simulink model "Copy_of_VTOLTiltrotor"  (R2024a)
settings: configuration reference "VTOLConfiguration" (kept outside this file)
undefined symbols (not defined in the file): airspeed, Battery, BCE12, BCE_Set_init, BMS_Controller_State, C, Cell10_P, Cell11_P, Cell12_P, Cell1_N, Cell1_P, Cell2_P, Cell3_P, Cell4_P, Cell5_P, Cell6_P, Cell7_P, Cell8_P, Cell9_P, Cell_Temperatures, Cell_Voltages, Charging_State, CityMission, control, controlParams, ControlSampleTime, CriticalTiltAngle, currentFactor, CV_Gain, ddx, ddy, ddz, Device_01, DiscIntNeverNeededParam, dx, dy, dz, Earth, env, F, F28379D_ADC_MaxCount, F28379D_ADC_Vmax, FixedWingMission, flightState, Foc_Ki_IxTcpu, Foc_Ki_S, Foc_Kp_I, Foc_Kp_S, fractalcoef, FSState, FWControlParams, HoverMission, I_cc, Ia_offset, Ib_offset, iniRoll, initPitch, iniYaw, IO334, IO334_DAC_Vmax ... (+55)
libraries: slrealtimeethercatlib x109, simulink x81, fl_lib x65, slpidlib x49, mcbcontrolslib x48, nesl_utility x43, speedgoatlib_hdlCoder_IO3xx x31, canmsglib x17, slrealtimeutilitieslib x13, mcbhdlplantlib x13, speedgoatlib_IO611 x12, dspstat3 x12
(part 1 of 20)
settings Model: DataDictionary=VTOLDynamicsData.sldd  Creator=The MathWorks, Inc.  LastModifiedBy=jatin.anand
settings ConfigSetRef: SourceName=VTOLConfiguration

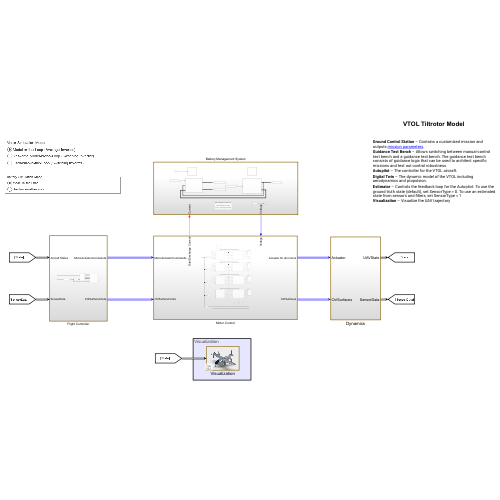
[thumbnail: Simulink's stored preview of the top-level diagram]
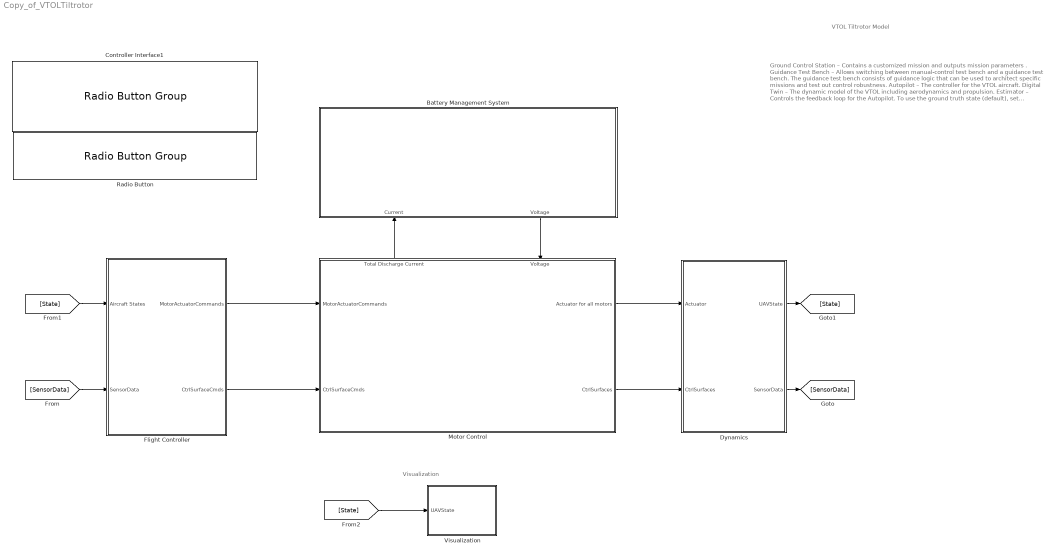
== system Copy_of_VTOLTiltrotor ==
  note: Ground Control Station – Contains a customized mission and outputs mission parameters .
      | Guidance Test Bench – Allows switching between manual-control test bench and a guidance test bench. The guidance test bench consists of guidance logic that can be used to architect specific missions and test out control robustness.
      | Autopilot – The controller for the VTOL aircraft.
      | Digital Twin – The dynamic model of the VTOL including aerodynamics and propulsion.
      | Estimator – Controls the feedback loop for the Autopilot. To use the ground truth state (default), set SensorType = 0. To use an estimated state from sensors and filters, set SensorType = 1
      | Visualization – Visualize the UAV trajectory
  note: VTOL Tiltrotor Model
  note: Visualization
  Battery Management System : Subsystem
      settings: PortSchema="{\"entries\":[{\"content\":{\"sides\":[{\"content\":{},\"type\":\"ConnectorPlacement.EquallySpacedRectSide\",\"uuid\":\"ad4822d7-5628-4510-88b7-b705ff74b914\"},{\"content\":{\"side\":\"RIGHT\"},\"type\":\"ConnectorPlacement.EquallySpacedRectSide\",\"uuid\":\"08045353-b32a-4841-afa7-c31ec693f3bd\"},{\"content\":{\"side\":\"TOP\"},\"type\":\"ConnectorPlacement.EquallySpacedRectSide\",\"uuid\":\"6a6533a3-371c-43cc-ab21-2cdd93971ace\"},{\"content\":{\"connectorIds\":[\"In1\",\"Out1\"],\"side\":\"BOTTOM\"},\"type\":\"ConnectorPlacement.EquallySpacedRectSide\",\"uuid\":\"23933915-aea2-4276-b64d-d3fc5163d9da\"}]},\"type\":\"ConnectorPlacement.EquallySpacedConnector\",\"uuid\":\"ad7e7a57-8abd-4902-b93b-ccdedcf72dce\"}],\"packageUris\":[\"http://schema.mathworks.com/mf0/Connector/R2020b\"],\"version\":\"1.0\"}"
  Controller Interface1 : RadioButtonGroup  LabelPosition=Hide  SelectedLabel=Model-in-the-Loop (Average Inverter)  ButtonGroupName=Motor Simulation Mode
      settings: Values={{'Model-in-the-Loop (Average Inverter)', 'Real-time Model-in-the-Loop (Switching Inverter)', 'Hardware-in-the-Loop (Switching Inverter)'}, [1 2 3]}
  Dynamics : Subsystem
  Flight Controller : Subsystem
  Motor Control : Subsystem
      settings: PortSchema="{\"entries\":[{\"content\":{\"sides\":[{\"content\":{\"connectorIds\":[\"In1\",\"In2\"]},\"type\":\"ConnectorPlacement.EquallySpacedRectSide\",\"uuid\":\"94b5e33d-15f7-4229-89dd-c5549510cb9d\"},{\"content\":{\"connectorIds\":[\"Out1\",\"Out2\"],\"side\":\"RIGHT\"},\"type\":\"ConnectorPlacement.EquallySpacedRectSide\",\"uuid\":\"879591cf-6d91-4a7e-b358-28ad8026a1fe\"},{\"content\":{\"connectorIds\":[\"Out3\",\"In3\"],\"side\":\"TOP\"},\"type\":\"ConnectorPlacement.EquallySpacedRectSide\",\"uuid\":\"fed77af4-f074-449a-8fce-c96eeb48edb7\"}]},\"type\":\"ConnectorPlacement.EquallySpacedConnector\",\"uuid\":\"f2702da8-edb1-45fe-ba32-a4867476937a\"}],\"packageUris\":[\"http://schema.mathworks.com/mf0/Connector/R2020b\"],\"version\":\"1.0\"}"
  Radio Button : RadioButtonGroup  LabelPosition=Hide  SelectedLabel=Model-in-the-Loop  ButtonGroupName=Battery Simulation Mode
      settings: Values={{'Model-in-the-Loop', 'Hardware-in-the-Loop'}, [0 1]}
  Visualization : Subsystem  Variant=on  VariantControl=Visualization
      mask Display: image('TiltrotorVisualization.PNG'); % Use "Edit Image" on toolstrip to change.
  wires:
  Dynamics/2(SensorData) -> [SensorData]
  Dynamics/1(UAVState) -> [State]
  [SensorData] -> Flight Controller/2(SensorData)
  [State] -> Flight Controller/1(Aircraft States)
  [State] -> Visualization/1(UAVState)
  Flight Controller/1(MotorActuatorCommands) -> Motor Control/1(MotorActuatorCommands)
  Flight Controller/2(CtrlSurfaceCmds) -> Motor Control/2(CtrlSurfaceCmds)
  Motor Control/1(Actuator for all motors) -> Dynamics/1(Actuator)
  Motor Control/2(CtrlSurfaces) -> Dynamics/2(CtrlSurfaces)
  Motor Control/3(Total Discharge Current) -> Battery Management System/1(Current)
  Battery Management System/1(Voltage) -> Motor Control/3(Voltage)

== system Copy_of_VTOLTiltrotor/Battery Management System ==
  note: Battery Management System HIL
      |
      | Reference application model
      | © 2007 - 2024 Speedgoat GmbH
  Current : Inport
  BMS : Subsystem  Variant=on  VariantControl=Choice
      mask Display: image('BMS.png'); % Use "Edit Image" on toolstrip to change.
  Battery : Subsystem
      mask Display: image('battery.png'); % Use "Edit Image" on toolstrip to change.
  Instrumentation : Subsystem
      mask Display: image('tunable.png'); % Use "Edit Image" on toolstrip to change.
  User Interface : Subsystem
      mask Display: image('UI.png'); % Use "Edit Image" on toolstrip to change.
  Voltage : Outport
  tag scope: Controller_Info=global, Controller_Output=global, Sensor_Values=global
  wires:
  [Current_Request] -> Battery/1(Current_Request)
  BMS/1(Controller_Info) -> [Controller_Info]  "Controller_Info"
  Battery/1(Sensor_Values) -> [Sensor_Values], BMS/2(Sensor_Values)
  [State_Request] -> BMS/1(State_Request)
  BMS/2(Controller_Output) -> [Controller_Output]  "Controller_Output"
  Current/1 -> Instrumentation/1(Current)
  [Voltage] -> Voltage/1
  connections:
  Battery/RConn1 -- BMS/LConn1

== system Copy_of_VTOLTiltrotor/Dynamics ==
  note: Forces and Moments - VTOL UAV plant model and weather model
      | 6DOF (Euler Angles Conversion) - Converts forces and moments from body to inertial frame
      | Ground Truth Bus - converts UAV States into bus
  Actuator : Inport
  CtrlSurfaces : Inport  Port=2
  6DOF (Euler Angles)1 : shared6dof/6DOF (Euler Angles)  units=Metric (MKS)  mtype=Fixed  rep=Euler Angles  xme_0=[xGround, yGround, zGround]  Vm_0=[vIni 0 0]  eul_0=[iniRoll initPitch iniYaw]  pm_0=[0 0 0]  mass_0=6.031  mass_e=0.5  mass_f=2.0  inertia=[uavParam.geom.Ixx 0 0; 0 uavParam.geom.Iyy 0; 0 0 uavParam.geom.Izz]  inertia_e=eye(3)  inertia_f=2*eye(3)  k_quat=1.0  vre_flag=on  abi_flag=on  aMode=0  xme_statename=''  Vm_statename=''  eul_statename=''  quat_statename=''  pm_statename=''  mass_statename=''
  Bus Selector : BusSelector  OutputSignals=RotorParameters.w1,RotorParameters.w2,RotorParameters.w3,RotorParameters.w4
  Force and Moments : Subsystem
  Ground Truth Bus : Subsystem
  Scope : Scope  NumInputPorts=4
  Terminator : Terminator
  Variant Subsystem : Subsystem  Variant=on  VariantControl=Choice
  UAVState : Outport
  SensorData : Outport  Port=2
  wires:
  Force and Moments/1(F) -> 6DOF (Euler Angles)1/1
  Force and Moments/2(M) -> 6DOF (Euler Angles)1/2
  Actuator/1 -> Force and Moments/1(Actuator)
  CtrlSurfaces/1 -> Force and Moments/2(CtrlSurfaces)
  6DOF (Euler Angles)1/1 -> Ground Truth Bus/1(Ve)  "Ve"
  6DOF (Euler Angles)1/2 -> Ground Truth Bus/2(Xe)  "Xe"
  6DOF (Euler Angles)1/3 -> Ground Truth Bus/3(Euler)  "Euler"
  6DOF (Euler Angles)1/4 -> Ground Truth Bus/4(DCMbe)  "DCMbe"
  6DOF (Euler Angles)1/5 -> Ground Truth Bus/5(Vb)  "Vb"
  6DOF (Euler Angles)1/6 -> Ground Truth Bus/6(pqr)  "pqr"
  6DOF (Euler Angles)1/7 -> Terminator/1
  6DOF (Euler Angles)1/8 -> Ground Truth Bus/7(Abb)  "Abb"
  Force and Moments/3(RotorParams) -> Ground Truth Bus/9(RotorParams)  "RotorParams"
  Force and Moments/4(AirData) -> Ground Truth Bus/10(AirData)
  Variant Subsystem/1(SensorData) -> SensorData/1
  6DOF (Euler Angles)1/9 -> Ground Truth Bus/8(Abe)
  Ground Truth Bus/1(Ground Truth) -> Bus Selector/1, UAVState/1, Force and Moments/3(States), Variant Subsystem/1(UAVStates)  "Ground Truth"
  Bus Selector/1 -> Scope/1  "<w1>"
  Bus Selector/2 -> Scope/2  "<w2>"
  Bus Selector/3 -> Scope/3  "<w3>"
  Bus Selector/4 -> Scope/4  "<w4>"

== system Copy_of_VTOLTiltrotor/Flight Controller ==
  Aircraft States : Inport
  SensorData : Inport  Port=2
  Autopilot : Subsystem
  Estimator : Subsystem  Variant=on
  Ground Control Station : Subsystem
  Guidance Test Bench : Subsystem
  MotorActuatorCommands : Outport
  CtrlSurfaceCmds : Outport  Port=2
  wires:
  Guidance Test Bench/3(AACSP) -> Autopilot/3(AAC)
  Estimator/1(EstimatedStates) -> Autopilot/6(EstimatedStates), Ground Control Station/1(UAVState)
  Ground Control Station/1(Global Mission) -> Guidance Test Bench/2(Global Mission)
  Guidance Test Bench/5(FlightMode) -> Autopilot/5(FlightMode)
  Guidance Test Bench/1(HoverSP) -> Autopilot/1(HoverCommands)
  Guidance Test Bench/2(FixedWingSP) -> Autopilot/2(FixedWingSP)
  SensorData/1 -> Estimator/1(SensorData)
  Guidance Test Bench/4(ctrlMode) -> Autopilot/4(CtrlMode)
  Autopilot/1(MotorActuatorCommands) -> MotorActuatorCommands/1
  Autopilot/2(CtrlSurfaceCmds) -> CtrlSurfaceCmds/1
  Aircraft States/1 -> Guidance Test Bench/1(Aircraft States)

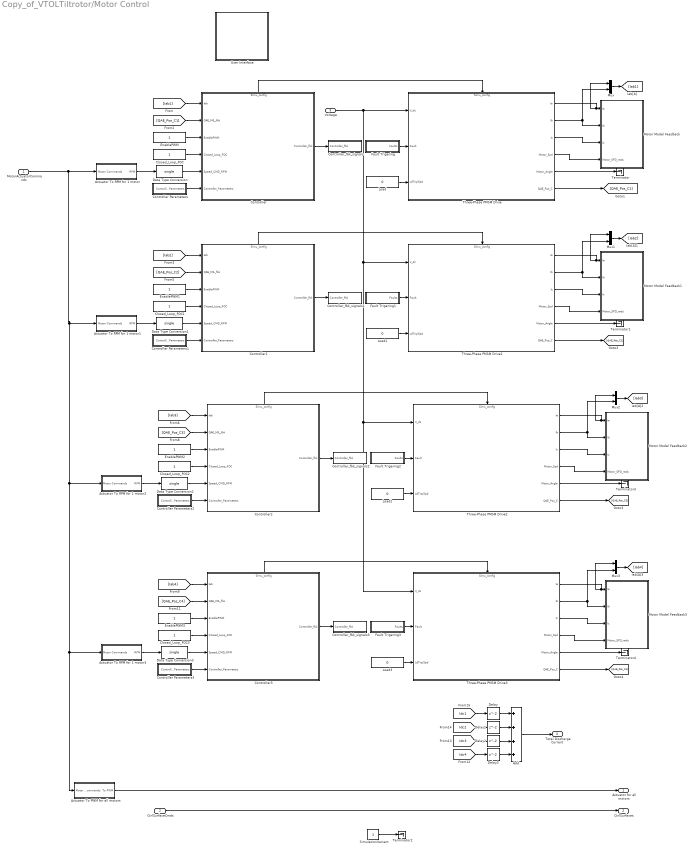
== system Copy_of_VTOLTiltrotor/Motor Control ==
  MotorActuatorCommands : Inport
  CtrlSurfaceCmds : Inport  Port=2
  Voltage : Inport  Port=3
  Actuator To PWM for all motors : Subsystem
  Actuator To RPM for 1 motor : Subsystem
  Actuator To RPM for 1 motor1 : Subsystem
  Actuator To RPM for 1 motor2 : Subsystem
  Actuator To RPM for 1 motor3 : Subsystem
  Add : Sum  Inputs=++++
  Closed_Loop_FOC{,1..3} (4 alike) : Constant  OutDataTypeStr=boolean  SampleTime=Ts_UI
  Controller : Subsystem  Variant=on  VariantControl=Choice
      settings: PortSchema="{\"entries\":[{\"content\":{\"sides\":[{\"content\":{\"connectorIds\":[\"In1\",\"In2\",\"In3\",\"In4\",\"In5\",\"In6\"]},\"type\":\"ConnectorPlacement.EquallySpacedRectSide\",\"uuid\":\"39f08c92-b87f-4f95-877f-fef0e466fbdb\"},{\"content\":{\"connectorIds\":[\"Out1\"],\"side\":\"RIGHT\"},\"type\":\"ConnectorPlacement.EquallySpacedRectSide\",\"uuid\":\"6fadd6f2-7db3-41c1-89a7-be1692c18c49\"},{\"content\":{\"connectorIds\":[\"Out2\"],\"side\":\"TOP\"},\"type\":\"ConnectorPlacement.EquallySpacedRectSide\",\"uuid\":\"aea4ee68-7094-4bdc-b416-2d8969306971\"}]},\"type\":\"ConnectorPlacement.EquallySpacedConnector\",\"uuid\":\"e129f01f-1291-4735-8ea4-164650c1b4f8\"}],\"packageUris\":[\"http://schema.mathworks.com/mf0/Connector/R2020b\"],\"version\":\"1.0\"}"
      mask Display: image('MCUMask.png');
  Controller Parameters : Subsystem
  Controller Parameters1 : Subsystem
  Controller Parameters2 : Subsystem
  Controller Parameters3 : Subsystem
  Controller1 : Subsystem  Variant=on  VariantControl=Choice
      settings: PortSchema="{\"entries\":[{\"content\":{\"sides\":[{\"content\":{\"connectorIds\":[\"In1\",\"In2\",\"In3\",\"In4\",\"In5\",\"In6\"]},\"type\":\"ConnectorPlacement.EquallySpacedRectSide\",\"uuid\":\"39f08c92-b87f-4f95-877f-fef0e466fbdb\"},{\"content\":{\"connectorIds\":[\"Out1\"],\"side\":\"RIGHT\"},\"type\":\"ConnectorPlacement.EquallySpacedRectSide\",\"uuid\":\"6fadd6f2-7db3-41c1-89a7-be1692c18c49\"},{\"content\":{\"connectorIds\":[\"Out2\"],\"side\":\"TOP\"},\"type\":\"ConnectorPlacement.EquallySpacedRectSide\",\"uuid\":\"aea4ee68-7094-4bdc-b416-2d8969306971\"}]},\"type\":\"ConnectorPlacement.EquallySpacedConnector\",\"uuid\":\"e129f01f-1291-4735-8ea4-164650c1b4f8\"}],\"packageUris\":[\"http://schema.mathworks.com/mf0/Connector/R2020b\"],\"version\":\"1.0\"}"
      mask Display: image('MCUMask.png');
  Controller2 : Subsystem  Variant=on  VariantControl=Choice
      settings: PortSchema="{\"entries\":[{\"content\":{\"sides\":[{\"content\":{\"connectorIds\":[\"In1\",\"In2\",\"In3\",\"In4\",\"In5\",\"In6\"]},\"type\":\"ConnectorPlacement.EquallySpacedRectSide\",\"uuid\":\"39f08c92-b87f-4f95-877f-fef0e466fbdb\"},{\"content\":{\"connectorIds\":[\"Out1\"],\"side\":\"RIGHT\"},\"type\":\"ConnectorPlacement.EquallySpacedRectSide\",\"uuid\":\"6fadd6f2-7db3-41c1-89a7-be1692c18c49\"},{\"content\":{\"connectorIds\":[\"Out2\"],\"side\":\"TOP\"},\"type\":\"ConnectorPlacement.EquallySpacedRectSide\",\"uuid\":\"aea4ee68-7094-4bdc-b416-2d8969306971\"}]},\"type\":\"ConnectorPlacement.EquallySpacedConnector\",\"uuid\":\"e129f01f-1291-4735-8ea4-164650c1b4f8\"}],\"packageUris\":[\"http://schema.mathworks.com/mf0/Connector/R2020b\"],\"version\":\"1.0\"}"
      mask Display: image('MCUMask.png');
  Controller3 : Subsystem  Variant=on  VariantControl=Choice
      settings: PortSchema="{\"entries\":[{\"content\":{\"sides\":[{\"content\":{\"connectorIds\":[\"In1\",\"In2\",\"In3\",\"In4\",\"In5\",\"In6\"]},\"type\":\"ConnectorPlacement.EquallySpacedRectSide\",\"uuid\":\"39f08c92-b87f-4f95-877f-fef0e466fbdb\"},{\"content\":{\"connectorIds\":[\"Out1\"],\"side\":\"RIGHT\"},\"type\":\"ConnectorPlacement.EquallySpacedRectSide\",\"uuid\":\"6fadd6f2-7db3-41c1-89a7-be1692c18c49\"},{\"content\":{\"connectorIds\":[\"Out2\"],\"side\":\"TOP\"},\"type\":\"ConnectorPlacement.EquallySpacedRectSide\",\"uuid\":\"aea4ee68-7094-4bdc-b416-2d8969306971\"}]},\"type\":\"ConnectorPlacement.EquallySpacedConnector\",\"uuid\":\"e129f01f-1291-4735-8ea4-164650c1b4f8\"}],\"packageUris\":[\"http://schema.mathworks.com/mf0/Connector/R2020b\"],\"version\":\"1.0\"}"
      mask Display: image('MCUMask.png');
  Controller_fbk_signals : Subsystem
  Controller_fbk_signals1 : Subsystem
  Controller_fbk_signals2 : Subsystem
  Controller_fbk_signals3 : Subsystem
  Data Type Conversion{,1..3} (4 alike) : DataTypeConversion  OutDataTypeStr=single  SaturateOnIntegerOverflow=off  RndMeth=Floor
  Delay{,1..3} (4 alike) : Delay
  EnablePWM{,1..3} (4 alike) : Constant  OutDataTypeStr=boolean  SampleTime=Ts_UI
  Fault Trigering : Subsystem
  Fault Trigering1 : Subsystem
  Fault Trigering2 : Subsystem
  Fault Trigering3 : Subsystem
  Load{,1..3} (4 alike) : Constant  Value=0  OutDataTypeStr=single
  Motor Model Feedback : Subsystem
  Motor Model Feedback1 : Subsystem
  Motor Model Feedback2 : Subsystem
  Motor Model Feedback3 : Subsystem
  Mux{,1..3} (4 alike) : Mux  Inputs=2
  SimulationVariant : Constant
  Terminator{,1..4} (5 alike) : Terminator
  Three-Phase PMSM Drive : Subsystem  Variant=on  VariantControl=Choice
      settings: PortSchema="{\"entries\":[{\"content\":{\"sides\":[{\"content\":{\"connectorIds\":[\"In1\",\"In2\",\"In3\"]},\"type\":\"ConnectorPlacement.EquallySpacedRectSide\",\"uuid\":\"be3bef0c-fa0d-49a9-8d81-4a9438f9f09e\"},{\"content\":{\"connectorIds\":[\"Out1\",\"Out2\",\"Out3\",\"Out4\",\"Out5\",\"Out6\"],\"side\":\"RIGHT\"},\"type\":\"ConnectorPlacement.EquallySpacedRectSide\",\"uuid\":\"a97c4291-bd47-47ae-a87a-e148291abc4a\"},{\"content\":{\"connectorIds\":[\"In4\"],\"side\":\"TOP\"},\"type\":\"ConnectorPlacement.EquallySpacedRectSide\",\"uuid\":\"93bcf0c4-5b44-4ac3-b6c3-6b4577237bd1\"}]},\"type\":\"ConnectorPlacement.EquallySpacedConnector\",\"uuid\":\"9c4ab161-5f4a-4191-8213-47b9045836c1\"}],\"packageUris\":[\"http://schema.mathworks.com/mf0/Connector/R2020b\"],\"version\":\"1.0\"}"
      mask Display: image('pmsmMask.png'); % Use "Edit Image" on toolstrip to change.
  Three-Phase PMSM Drive1 : Subsystem  Variant=on  VariantControl=Choice
      settings: PortSchema="{\"entries\":[{\"content\":{\"sides\":[{\"content\":{\"connectorIds\":[\"In1\",\"In2\",\"In3\"]},\"type\":\"ConnectorPlacement.EquallySpacedRectSide\",\"uuid\":\"be3bef0c-fa0d-49a9-8d81-4a9438f9f09e\"},{\"content\":{\"connectorIds\":[\"Out1\",\"Out2\",\"Out3\",\"Out4\",\"Out5\",\"Out6\"],\"side\":\"RIGHT\"},\"type\":\"ConnectorPlacement.EquallySpacedRectSide\",\"uuid\":\"a97c4291-bd47-47ae-a87a-e148291abc4a\"},{\"content\":{\"connectorIds\":[\"In4\"],\"side\":\"TOP\"},\"type\":\"ConnectorPlacement.EquallySpacedRectSide\",\"uuid\":\"93bcf0c4-5b44-4ac3-b6c3-6b4577237bd1\"}]},\"type\":\"ConnectorPlacement.EquallySpacedConnector\",\"uuid\":\"9c4ab161-5f4a-4191-8213-47b9045836c1\"}],\"packageUris\":[\"http://schema.mathworks.com/mf0/Connector/R2020b\"],\"version\":\"1.0\"}"
      mask Display: image('pmsmMask.png'); % Use "Edit Image" on toolstrip to change.
  Three-Phase PMSM Drive2 : Subsystem  Variant=on  VariantControl=Choice
      settings: PortSchema="{\"entries\":[{\"content\":{\"sides\":[{\"content\":{\"connectorIds\":[\"In1\",\"In2\",\"In3\"]},\"type\":\"ConnectorPlacement.EquallySpacedRectSide\",\"uuid\":\"be3bef0c-fa0d-49a9-8d81-4a9438f9f09e\"},{\"content\":{\"connectorIds\":[\"Out1\",\"Out2\",\"Out3\",\"Out4\",\"Out5\",\"Out6\"],\"side\":\"RIGHT\"},\"type\":\"ConnectorPlacement.EquallySpacedRectSide\",\"uuid\":\"a97c4291-bd47-47ae-a87a-e148291abc4a\"},{\"content\":{\"connectorIds\":[\"In4\"],\"side\":\"TOP\"},\"type\":\"ConnectorPlacement.EquallySpacedRectSide\",\"uuid\":\"93bcf0c4-5b44-4ac3-b6c3-6b4577237bd1\"}]},\"type\":\"ConnectorPlacement.EquallySpacedConnector\",\"uuid\":\"9c4ab161-5f4a-4191-8213-47b9045836c1\"}],\"packageUris\":[\"http://schema.mathworks.com/mf0/Connector/R2020b\"],\"version\":\"1.0\"}"
      mask Display: image('pmsmMask.png'); % Use "Edit Image" on toolstrip to change.
  Three-Phase PMSM Drive3 : Subsystem  Variant=on  VariantControl=Choice
      settings: PortSchema="{\"entries\":[{\"content\":{\"sides\":[{\"content\":{\"connectorIds\":[\"In1\",\"In2\",\"In3\"]},\"type\":\"ConnectorPlacement.EquallySpacedRectSide\",\"uuid\":\"be3bef0c-fa0d-49a9-8d81-4a9438f9f09e\"},{\"content\":{\"connectorIds\":[\"Out1\",\"Out2\",\"Out3\",\"Out4\",\"Out5\",\"Out6\"],\"side\":\"RIGHT\"},\"type\":\"ConnectorPlacement.EquallySpacedRectSide\",\"uuid\":\"a97c4291-bd47-47ae-a87a-e148291abc4a\"},{\"content\":{\"connectorIds\":[\"In4\"],\"side\":\"TOP\"},\"type\":\"ConnectorPlacement.EquallySpacedRectSide\",\"uuid\":\"93bcf0c4-5b44-4ac3-b6c3-6b4577237bd1\"}]},\"type\":\"ConnectorPlacement.EquallySpacedConnector\",\"uuid\":\"9c4ab161-5f4a-4191-8213-47b9045836c1\"}],\"packageUris\":[\"http://schema.mathworks.com/mf0/Connector/R2020b\"],\"version\":\"1.0\"}"
      mask Display: image('pmsmMask.png'); % Use "Edit Image" on toolstrip to change.
  User Interface : Subsystem
      mask Display: image('UIMask.png');
  Actuator for all motors : Outport
  CtrlSurfaces : Outport  Port=2
  Total Discharge Current : Outport  Port=3
  wires:
  CtrlSurfaceCmds/1 -> CtrlSurfaces/1
  SimulationVariant/1 -> Terminator2/1
  Controller/1(Controller_fbk) -> Controller_fbk_signals/1(Controller_fbk)
  [Iab1] -> Controller/1(Iab)
  Three-Phase PMSM Drive/4(Motor_Spd) -> Motor Model Feedback/4(Motor_SPD_rads)
  Three-Phase PMSM Drive/3(Ic) -> Motor Model Feedback/3(Ic)
  [QAE_Pos_C1] -> Controller/2(QAE_MIL_fbk)
  Three-Phase PMSM Drive/2(Ib) -> Mux/2, Motor Model Feedback/2(Ib)
  Controller Parameters/1(Controller Parameters) -> Controller/6(Controller_Parameters)
  Three-Phase PMSM Drive/1(Ia) -> Mux/1, Motor Model Feedback/1(Ia)
  EnablePWM/1 -> Controller/3(EnablePWM)
  Three-Phase PMSM Drive/5(Motor_Angle) -> Terminator/1
  Load/1 -> Three-Phase PMSM Drive/3(LdTrq/Spd)
  Mux/1 -> [Iab1]
  Closed_Loop_FOC/1 -> Controller/4(Closed_Loop_FOC)
  Fault Trigering/1(Faults) -> Three-Phase PMSM Drive/2(Fault)
  Three-Phase PMSM Drive/6(QAE_Pos_C) -> [QAE_Pos_C1]
  Controller/2(Simu_config) -> Three-Phase PMSM Drive/4(Simu_config)
  Actuator To RPM for 1 motor/1(RPM) -> Data Type Conversion/1
  Actuator To PWM for all motors/1(To PWM) -> Actuator for all motors/1
  Data Type Conversion/1 -> Controller/5(Speed_CMD_RPM)
  Three-Phase PMSM Drive1/5(Motor_Angle) -> Terminator1/1
  Load1/1 -> Three-Phase PMSM Drive1/3(LdTrq/Spd)
  Three-Phase PMSM Drive1/4(Motor_Spd) -> Motor Model Feedback1/4(Motor_SPD_rads)
  [Iab2] -> Controller1/1(Iab)
  Three-Phase PMSM Drive1/3(Ic) -> Motor Model Feedback1/3(Ic)
  Mux1/1 -> [Iab2]
  Three-Phase PMSM Drive1/2(Ib) -> Mux1/2, Motor Model Feedback1/2(Ib)
  Data Type Conversion1/1 -> Controller1/5(Speed_CMD_RPM)
  Controller Parameters1/1(Controller Parameters) -> Controller1/6(Controller_Parameters)
  Three-Phase PMSM Drive1/6(QAE_Pos_C) -> [QAE_Pos_C2]
  [QAE_Pos_C2] -> Controller1/2(QAE_MIL_fbk)
  Controller1/2(Simu_config) -> Three-Phase PMSM Drive1/4(Simu_config)
  Fault Trigering1/1(Faults) -> Three-Phase PMSM Drive1/2(Fault)
  EnablePWM1/1 -> Controller1/3(EnablePWM)
  Closed_Loop_FOC1/1 -> Controller1/4(Closed_Loop_FOC)
  Controller1/1(Controller_fbk) -> Controller_fbk_signals1/1(Controller_fbk)
  Three-Phase PMSM Drive1/1(Ia) -> Mux1/1, Motor Model Feedback1/1(Ia)
  Actuator To RPM for 1 motor1/1(RPM) -> Data Type Conversion1/1
  Controller2/1(Controller_fbk) -> Controller_fbk_signals2/1(Controller_fbk)
  Closed_Loop_FOC2/1 -> Controller2/4(Closed_Loop_FOC)
  Fault Trigering2/1(Faults) -> Three-Phase PMSM Drive2/2(Fault)
  Three-Phase PMSM Drive2/6(QAE_Pos_C) -> [QAE_Pos_C3]
  Actuator To RPM for 1 motor2/1(RPM) -> Data Type Conversion2/1
  Controller Parameters2/1(Controller Parameters) -> Controller2/6(Controller_Parameters)
  Data Type Conversion2/1 -> Controller2/5(Speed_CMD_RPM)
  Three-Phase PMSM Drive2/1(Ia) -> Mux2/1, Motor Model Feedback2/1(Ia)
  Controller2/2(Simu_config) -> Three-Phase PMSM Drive2/4(Simu_config)
  [QAE_Pos_C3] -> Controller2/2(QAE_MIL_fbk)
  Three-Phase PMSM Drive2/2(Ib) -> Mux2/2, Motor Model Feedback2/2(Ib)
  [Iab3] -> Controller2/1(Iab)
  Three-Phase PMSM Drive2/3(Ic) -> Motor Model Feedback2/3(Ic)
  Load2/1 -> Three-Phase PMSM Drive2/3(LdTrq/Spd)
  Three-Phase PMSM Drive2/4(Motor_Spd) -> Motor Model Feedback2/4(Motor_SPD_rads)
  Mux2/1 -> [Iab3]
  Voltage/1 -> Three-Phase PMSM Drive3/1(V_dc), Three-Phase PMSM Drive2/1(V_dc), Three-Phase PMSM Drive1/1(V_dc), Three-Phase PMSM Drive/1(V_dc)
  EnablePWM2/1 -> Controller2/3(EnablePWM)
  Three-Phase PMSM Drive2/5(Motor_Angle) -> Terminator3/1
  Controller3/1(Controller_fbk) -> Controller_fbk_signals3/1(Controller_fbk)
  Closed_Loop_FOC3/1 -> Controller3/4(Closed_Loop_FOC)
  Fault Trigering3/1(Faults) -> Three-Phase PMSM Drive3/2(Fault)
  Three-Phase PMSM Drive3/6(QAE_Pos_C) -> [QAE_Pos_C4]
  Actuator To RPM for 1 motor3/1(RPM) -> Data Type Conversion3/1
  Controller Parameters3/1(Controller Parameters) -> Controller3/6(Controller_Parameters)
  Data Type Conversion3/1 -> Controller3/5(Speed_CMD_RPM)
  Three-Phase PMSM Drive3/1(Ia) -> Mux3/1, Motor Model Feedback3/1(Ia)
  Controller3/2(Simu_config) -> Three-Phase PMSM Drive3/4(Simu_config)
  [QAE_Pos_C4] -> Controller3/2(QAE_MIL_fbk)
  Three-Phase PMSM Drive3/2(Ib) -> Mux3/2, Motor Model Feedback3/2(Ib)
  [Iab4] -> Controller3/1(Iab)
  Three-Phase PMSM Drive3/3(Ic) -> Motor Model Feedback3/3(Ic)
  Load3/1 -> Three-Phase PMSM Drive3/3(LdTrq/Spd)
  Three-Phase PMSM Drive3/4(Motor_Spd) -> Motor Model Feedback3/4(Motor_SPD_rads)
  Mux3/1 -> [Iab4]
  EnablePWM3/1 -> Controller3/3(EnablePWM)
  Three-Phase PMSM Drive3/5(Motor_Angle) -> Terminator4/1
  MotorActuatorCommands/1 -> Actuator To RPM for 1 motor1/1(Motor Commands), Actuator To RPM for 1 motor2/1(Motor Commands), Actuator To RPM for 1 motor3/1(Motor Commands), Actuator To PWM for all motors/1(Motor Commands), Actuator To RPM for 1 motor/1(Motor Commands)
  [Idc4] -> Delay3/1
  [Idc3] -> Delay2/1
  [Idc2] -> Delay1/1
  [Idc1] -> Delay/1
  Add/1 -> Total Discharge Current/1
  Delay/1 -> Add/1
  Delay1/1 -> Add/2
  Delay2/1 -> Add/3
  Delay3/1 -> Add/4

== system Copy_of_VTOLTiltrotor/Visualization ==
  UAVState : Inport
  No Visualization : Subsystem  VariantControl=Visualization==0
  Photorealistic : Subsystem  VariantControl=Visualization==2
  Visualization : Subsystem  VariantControl=Visualization==1

== system Copy_of_VTOLTiltrotor/Battery Management System/BMS ==
  State_Request : Inport
  Sensor_Values : Inport  Port=2
  HIL : Subsystem  VariantControl=strcmp(get_param(['VTOLTiltrotor/Battery Management System/Instrumentation/Simulation_Profile_Value'], 'Value'),'1')
  MIL : Subsystem  VariantControl=strcmp(get_param(['VTOLTiltrotor/Battery Management System/Instrumentation/Simulation_Profile_Value'], 'Value'),'0')
  Cells : PMIOPort  Side=Left
  Controller_Info : Outport
  Controller_Output : Outport  Port=2

== system Copy_of_VTOLTiltrotor/Battery Management System/Battery ==
  Current_Request : Inport
  Battery Pack : Subsystem
  Bus Creator : BusCreator  Inputs=4  OutDataTypeStr=Bus: Sensor_Values  NonVirtualBus=on
      settings: InheritFromInputs=off
  Bypass : Subsystem
  Data Type Conversion{,1..3} (4 alike) : DataTypeConversion  OutDataTypeStr=single  SaturateOnIntegerOverflow=off  RndMeth=Floor
  Electrical Interface : Subsystem
  HW Interface : Subsystem  Variant=on  VariantControl=Choice
  Rate Transition1 : RateTransition  OutPortSampleTime=ts_system
  Cells : PMIOPort  Side=Right
  Sensor_Values : Outport
  tag scope: Cells_SOCs=global
  wires:
  Current_Request/1 -> Rate Transition1/1
  Electrical Interface/1(Pack_Current) -> Data Type Conversion2/1
  Electrical Interface/2(Pack_Voltage) -> Data Type Conversion1/1
  Data Type Conversion/1 -> Bus Creator/1  "Cell_Voltages"
  Data Type Conversion1/1 -> Bus Creator/4  "Pack_Voltage"
  Data Type Conversion2/1 -> Bus Creator/3  "Pack_Current"
  Data Type Conversion3/1 -> Bus Creator/2  "Cell_Temperatures"
  [Ambient_Temperature_User] -> Battery Pack/1(Ambient_Temperature)
  Battery Pack/1(Cell_Voltages) -> Data Type Conversion/1
  Battery Pack/2(Cell_Temperatures) -> Data Type Conversion3/1
  Battery Pack/3(Cell_SOCs) -> [Cells_SOCs]  "Cell_SOCs"
  Bus Creator/1 -> Bypass/1(IN)
  HW Interface/1(Sensor_Values_Real) -> Sensor_Values/1
  Rate Transition1/1 -> Electrical Interface/1(Current_Request)
  Bypass/1(OUT) -> HW Interface/1(Sensor_Values_Sim)
  [Short_Circuits_User] -> Battery Pack/2(Short_Circuits)
  connections:
  Battery Pack/RConn1 -- Electrical Interface/LConn1
  Battery Pack/RConn2 -- Electrical Interface/LConn2
  Battery Pack/RConn3 -- HW Interface/LConn1
  HW Interface/RConn1 -- Cells/RConn1

== system Copy_of_VTOLTiltrotor/Battery Management System/Instrumentation ==
  Current : Inport
  Ambient_Temperature : Constant  Value=25
  Celsius_to_Kelvin : Subsystem
  Constant1 : Constant
  Current Control : Subsystem
  Current_ : Constant  Value=-20
  Display : Display
  Instrumented Signals : Subsystem
  Simulation_Profile_Value : Constant  Value=0
  State_Request : simulink/Sources/Enumerated Constant  OutDataTypeStr=Enum: SRE  Value=SRE.Standby  SampleTime=inf
  Terminator4 : Terminator
  tag scope: Ambient_Temperature_User=global, Current_Request=global, Open_Circuits_User=global, Short_Circuits_User=global, State_Request=global
  wires:
  Celsius_to_Kelvin/1(K) -> [Ambient_Temperature_User]
  Ambient_Temperature/1 -> Celsius_to_Kelvin/1(C)
  Constant1/1 -> Current Control/2(Current_Request_User_Bypass)
  Current Control/1(Current_Request) -> [Current_Request]  "Pack_Current_Request"
  State_Request/1 -> [State_Request]
  [Controller_Output] -> Instrumented Signals/1(Controller_Output), Current Control/4(Controller_Output)
  [Controller_Info] -> Instrumented Signals/2(Controller_Info), Current Control/3(Controller_Info)
  [Sensor_Values] -> Instrumented Signals/3(Sensor_Values)
  [Balancing_Currents] -> Instrumented Signals/4(Balancing_Currents)
  [Cells_SOCs] -> Instrumented Signals/5(Cells_SOCs)
  Instrumented Signals/1(Short-Circuits) -> [Short_Circuits_User]
  Instrumented Signals/2(Open-Circuits) -> [Open_Circuits_User]
  Simulation_Profile_Value/1 -> Terminator4/1
  Current/1 -> Display/1, Current Control/1(Current_Request_User)
